simulink model "AM_EB_1"  (R2024a)
settings: Solver=VariableStepAuto  StartTime=0.0  StopTime=10.0  RelTol=1e-3
settings Model: Creator=Braan  LastModifiedBy=Braan

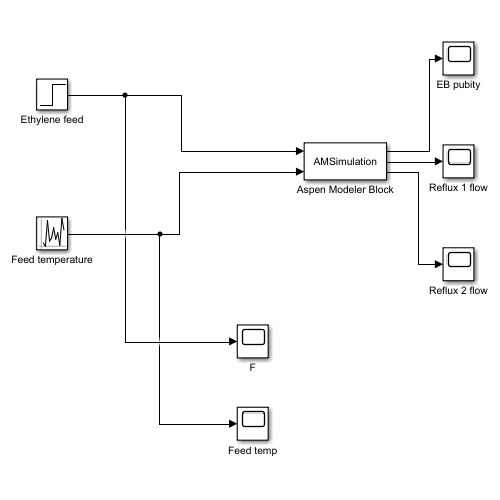
[thumbnail: Simulink's stored preview of the top-level diagram]
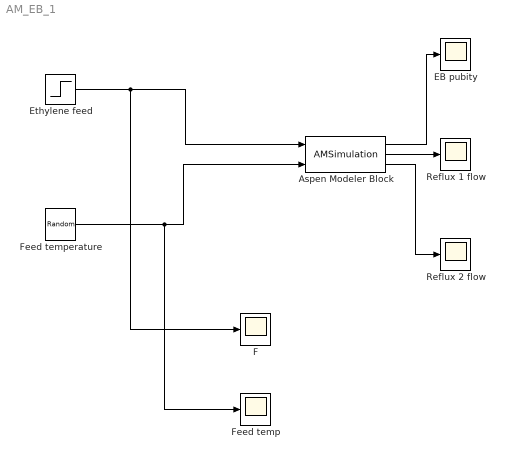
== system AM_EB_1 ==
  Aspen Modeler Block : M-S-Function  LoadFcn=|  FunctionName=AMSimulation  Parameters="'C:\\git\\master_project\\Aspen_files\\Ethyl Benzene\\Ethyl Benzene\\EB.dynf','AD Application',2,'ETHY_FC.SPRemote|kmol/hr\\S_ETHY.T|C',3,'STREAMS(\"S13\").Zmn(\"EB\")|kg/kg\\STREAMS(\"TOT\").F|kmol/hr\\STREAMS(\"S19\").F|kmol/hr',true,true,true"
      | LoadModel=actxserver('AMSimulation.Control');                 
      | invoke(LoadModel,'LoadModel',get_param(gcb,'Parameters'),pwd);
      | LoadModel.delete;
      | rehash;
      settings: DeleteFcn=|
      | CloseModel=actxserver('AMSimulation.Control');
      | invoke(CloseModel,'CloseModel',get_param(gcb,'Parameters'));
      | CloseModel.delete;
      settings: OpenFcn=|
      | SetupGUI=actxserver('AMSimulation.Setup');
      | NewParam=invoke(SetupGUI,'SetupModel',get_param(gcb,'Parameters'),pwd,get_param(gcb,'Name'));
      | set_param(gcb,'Parameters',NewParam);
      | SetupGUI.delete;
  EB pubity : Scope
  Ethylene feed : Step  Before=630.6  After=639.6*1.05  SampleTime=0
  F : Scope
  Feed temp : Scope
  Feed temperature : UniformRandomNumber  Minimum=44  Maximum=48  Seed=1  SampleTime=0.1
  Reflux 1 flow : Scope
  Reflux 2 flow : Scope
  wires:
  Ethylene feed/1 -> F/1, Aspen Modeler Block/1
  Feed temperature/1 -> Feed temp/1, Aspen Modeler Block/2
  Aspen Modeler Block/3 -> Reflux 2 flow/1
  Aspen Modeler Block/2 -> Reflux 1 flow/1
  Aspen Modeler Block/1 -> EB pubity/1
